simulink model "m02_PMSM_HDL"  (R2023b)
settings: Solver=FixedStepDiscrete  StartTime=0.0  StopTime=0.6  RelTol=1e-3  AbsTol=1e-3
PreLoadFcn:
  | control_data;
  | pmsm_data;
  | 
  | avgFactor = 1;
undefined symbols (not defined in the file): ee_sli_rtmsupport, f1478573793584, f1859323186544, fsw, gcbh, J, Ld, Lq, N, PM, Pmax, Tmax, Ts, Tsc
libraries: hdlssclib x24, simulink x8, SimscapeFPGAHIL_lib x6, fpga_utils_lib x5, hdlsllib x4, eeTransforms x2, eePwmGeneratorTwoLevel x1, eePmsmCurrentController x1, eePmsmCurrentReferenceGen x1, eeVelocityController x1
(part 1 of 3)
Description:
  | Three-Phase PMSM Drive
settings Model: DataTypeOverride=Off  SimulationMode=accelerator  Creator=The MathWorks, Inc.  LastModifiedBy=promero
settings SolverCC: AutoScaleAbsTol=off  MaxConsecutiveMinStep=2  ZeroCrossAlgorithm=Adaptive  AlgebraicLoopSolver=TrustRegion  MaxZcPerStep=1
settings DataIOCC: MaxDataPoints=690000  SaveOutput=off  DSMLogging=off  SaveTime=off
settings OptimizationCC: BlockReduction=off  ConditionallyExecuteInputs=off  DefaultParameterBehavior=Inlined  InheritOutputTypeSmallerThanSingle=on  ReuseModelBlockBuffer=off  LifeSpan=inf
settings DebuggingCC: AlgebraicLoopMsg=error  UnderspecifiedInitializationDetection=Classic  MergeDetectMultiDrivingBlocksExec=none  MaxConsecutiveZCsMsg=none  IgnoredZcDiagnostic=none  InheritedTsInSrcMsg=none  SingleTaskRateTransMsg=error  UnconnectedInputMsg=warning  UnconnectedOutputMsg=warning  UnconnectedLineMsg=warning  AllowSymbolicDim=off  PregeneratedLibrarySubsystemCodeDiagnostic=none  SFUnexpectedBacktrackingDiag=warning  SFNoUnconditionalDefaultTransitionDiag=warning  SFExecutionAtInitializationDiag=none  ArithmeticOperatorsInVariantConditions=warning
settings HardwareCC: ProdBitPerPointer=32  ProdBitPerSizeT=32  ProdBitPerPtrDiffT=32  ProdLargestAtomicFloat=None  ProdIntDivRoundTo=Undefined  ProdEndianess=Unspecified  ProdWordSize=32  ProdHWDeviceType=ASIC/FPGA->ASIC/FPGA  TargetBitPerPointer=64  TargetBitPerSizeT=64  TargetBitPerPtrDiffT=64  TargetLongLongMode=on  TargetIntDivRoundTo=Zero  TargetEndianess=LittleEndian  TargetWordSize=64  TargetHWDeviceType=Custom Processor->MATLAB Host Computer  ProdEqTarget=off
settings ModelReferenceCC: EnableRefExpFcnMdlSchedulingChecks=on  PropagateSignalLabelsOutOfModel=off
settings SFSimCC: SimUseLocalCustomCode=off
settings RTWCC: RTWUseLocalCustomCode=off  DLArmComputeVersion=19.05
settings CodeAppCC: StateflowObjectComments=on
settings GRTTargetCC: TargetLangStandard=C89/C90 (ANSI)
settings ConfigComp: CovMetricSettings=dw  CovSaveCumulativeToWorkspaceVar=on  CovSaveSingleToWorkspaceVar=on  CovExternalEMLEnable=off  CovSFcnEnable=off
settings SimscapeCC: SimscapeLogSimulationStatistics=on  SimscapeLogName=simlog_ee_pmsm_drive  SimscapeLogDataHistory=690000

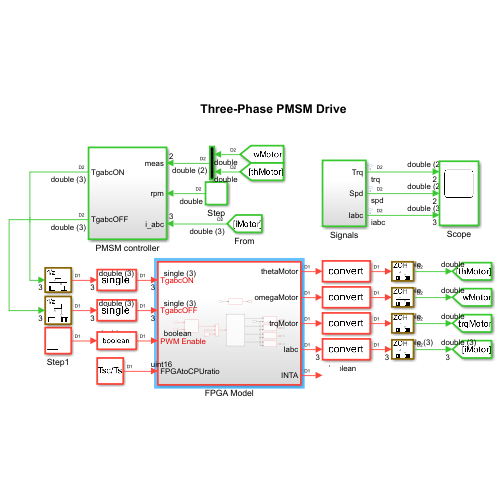
[thumbnail: Simulink's stored preview of the top-level diagram]
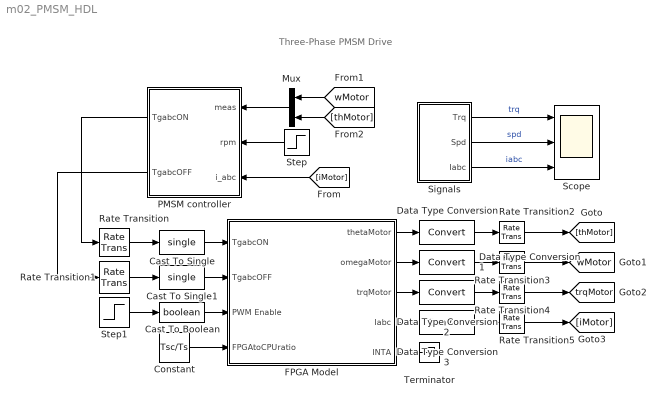
== system m02_PMSM_HDL ==
  note: Three-Phase PMSM Drive
  Cast To Boolean : DataTypeConversion  OutDataTypeStr=boolean  SaturateOnIntegerOverflow=off  RndMeth=Floor
  Cast To Single : DataTypeConversion  OutDataTypeStr=single  SaturateOnIntegerOverflow=off  RndMeth=Floor
  Cast To Single1 : DataTypeConversion  OutDataTypeStr=single  SaturateOnIntegerOverflow=off  RndMeth=Floor
  Constant : Constant  Value=Tsc/Ts  OutDataTypeStr=uint16  SampleTime=-1
  Data Type Conversion{,1..3} (4 alike) : DataTypeConversion  SaturateOnIntegerOverflow=off  RndMeth=Floor
  FPGA Model : Subsystem
  Mux : Mux  Inputs=2
  PMSM controller : Subsystem
  Rate Transition : RateTransition  OutPortSampleTime=Ts
  Rate Transition1 : RateTransition  OutPortSampleTime=Ts
  Rate Transition{2..5} (4 alike) : RateTransition  OutPortSampleTime=Tsc
  Scope : Scope  NumInputPorts=3
  "Signals " : Subsystem
  Step : Step  Time=0.1  After=500  SampleTime=Tsc
  Step1 : Step  Time=1e-4
  Terminator : Terminator
  tag scope: trqMotor=global, wMotor=global
  wires:
  "Signals "/2(Spd) -> Scope/2  "spd"
  "Signals "/1(Trq) -> Scope/1  "trq"
  "Signals "/3(Iabc) -> Scope/3  "iabc"
  Step/1 -> PMSM controller/2(rpm)
  Mux/1 -> PMSM controller/1(meas)
  [iMotor] -> PMSM controller/3(i_abc)
  PMSM controller/1(TgabcON) -> Rate Transition/1
  PMSM controller/2(TgabcOFF) -> Rate Transition1/1
  Step1/1 -> Cast To Boolean/1
  FPGA Model/1(thetaMotor) -> Data Type Conversion/1
  FPGA Model/2(omegaMotor) -> Data Type Conversion1/1
  FPGA Model/3(trqMotor) -> Data Type Conversion2/1
  FPGA Model/4(Iabc) -> Data Type Conversion3/1
  Data Type Conversion2/1 -> Rate Transition4/1
  Data Type Conversion3/1 -> Rate Transition5/1
  Data Type Conversion1/1 -> Rate Transition3/1
  Data Type Conversion/1 -> Rate Transition2/1
  [wMotor] -> Mux/1
  [thMotor] -> Mux/2
  Cast To Single/1 -> FPGA Model/1(TgabcON)
  Cast To Single1/1 -> FPGA Model/2(TgabcOFF)
  Cast To Boolean/1 -> FPGA Model/3(PWM Enable)
  Rate Transition/1 -> Cast To Single/1
  Rate Transition1/1 -> Cast To Single1/1
  Rate Transition2/1 -> [thMotor]
  Rate Transition3/1 -> [wMotor]
  Rate Transition4/1 -> [trqMotor]
  Rate Transition5/1 -> [iMotor]
  Constant/1 -> FPGA Model/4(FPGAtoCPUratio)
  FPGA Model/5(INTA) -> Terminator/1

== system m02_PMSM_HDL/FPGA Model ==
  TgabcON : Inport
  TgabcOFF : Inport  Port=2
  PWM Enable : Inport  Port=3
  FPGAtoCPUratio : Inport  Port=4
  Constant : Constant  Value=[0,1,0,1,0,1]  OutDataTypeStr=boolean  SampleTime=-1
  FPGAtoCPUratio1 : InportShadow  Port=4
  HDL Moving Average Tunable{,1..3} (4 alike) : fpga_utils_lib/HDL Moving Average Tunable  SystemSampleTime=-1  VariantActivationTime=update diagram  AllowFlexibleInterface=on  Latency=0  AutoFrameSizeCalculation=off
  HDL Plant : Subsystem  Variant=on  VariantControlMode=label  VariantControl=Pejovic HDL Plant  LabelModeActiveChoice=Pejovic
  Interrupt : fpga_utils_lib/Interrupt  SystemSampleTime=-1  VariantActivationTime=update diagram  AllowFlexibleInterface=on  Latency=0  AutoFrameSizeCalculation=off
  PWM Gate Signal Generator : Subsystem  Variant=on  VariantControlMode=label  VariantControl=Choice  LabelModeActiveChoice=hdlVar
  Switch : Switch  Criteria=u2 ~= 0  SaturateOnIntegerOverflow=off
  thetaMotor : Outport  OutDataTypeStr=single
  omegaMotor : Outport  Port=2  OutDataTypeStr=single
  trqMotor : Outport  Port=3  OutDataTypeStr=single
  Iabc : Outport  Port=4  OutDataTypeStr=single
  INTA : Outport  Port=5
  wires:
  Constant/1 -> Switch/3
  PWM Enable/1 -> Switch/2
  TgabcON/1 -> PWM Gate Signal Generator/1(TgabcON)
  TgabcOFF/1 -> PWM Gate Signal Generator/2(TgabcOFF)
  PWM Gate Signal Generator/1(g) -> Switch/1
  HDL Moving Average Tunable/1 -> thetaMotor/1
  HDL Moving Average Tunable1/1 -> omegaMotor/1
  HDL Moving Average Tunable2/1 -> trqMotor/1
  HDL Moving Average Tunable3/1 -> Iabc/1
  FPGAtoCPUratio/1 -> HDL Moving Average Tunable3/2, HDL Moving Average Tunable2/2, HDL Moving Average Tunable1/2, HDL Moving Average Tunable/2
  Interrupt/1 -> INTA/1
  FPGAtoCPUratio1/1 -> Interrupt/1
  Switch/1 -> HDL Plant/1(In1)
  HDL Plant/1(thetaMotor) -> HDL Moving Average Tunable/1
  HDL Plant/2(omegaMotor) -> HDL Moving Average Tunable1/1
  HDL Plant/3(trqMotor) -> HDL Moving Average Tunable2/1
  HDL Plant/4(Iabc) -> HDL Moving Average Tunable3/1

== system m02_PMSM_HDL/PMSM controller ==
  meas : Inport
  rpm : Inport  Port=2
  i_abc : Inport  Port=3
  Bus Selector : BusSelector  OutputSignals=iabc [A],Reference,TqRef [N*m]
  Demux1 : Demux  Outputs=2
  PMSM Field-Oriented Control : Subsystem  AncestorBlock=eePmsmFieldOrientedControl/PMSM Field-Oriented Control  LoadFcn=ee_sli_rtmsupport( 'loadfcn', gcbh );  mask(PMSM Field-Oriented Control){winding_type=Wye-wound, CtrlMode=Velocity control, Vnom=48, Pmax=Pmax, Tmax=Tmax*1.5, p=N, Vdc_on=10, Ts=Ts, Tsc=Tsc, CtrlType=PI control, Kp_w=60, Ki_w=300*2, Kv_w=1, Kaw_w=1000, RefType=Zero d-axis control, rpmVec=[0, 3000], TqVec=[-100, 0, 100], VdcVec=[300, 350], PWMMode=SPWM: sinusoidal PWM, ModFactor=1, idMatrix=zeros(2,3,2), iqMatrix=zeros(2,3,2), psim=PM, Ld=0.00024, Lq=0.00029, Rs=0.01, AxisAlignment=Q-axis, Kp_id=0.1, Ki_id=10, Kaw_id=1000, Kp_iq=0.1, Ki_iq=10, Kaw_iq=1000, AxisPrio=Q-axis, ActZC=off, ActFF=on, ParamTypeFF=Constant parameters, LdFF=Ld, LqFF=Lq, psimFF=PM, idVect=[-200, 0, 200], iqVect=[-200, 0, 200], LdMatrix=0.0002 * ones(3, 3), LqMatrix=0.0002 * ones(3, 3), psimMatrix=0.04 * ones(3, 3), CPWMMode=SPWM: sinusoidal PWM, SamplingMode=Natural, fsw=fsw}
      mask prompts: winding_type "physmod:ee:library:comments:control:eePmsmFieldOrientedControl:WindingType_MP"; CtrlMode "physmod:ee:library:comments:control:eePmsmFieldOrientedControl:ControlMode_MP"; Vnom "physmod:ee:library:comments:control:eePmsmFieldOrientedControl:NominalDclinkVoltageV_MP"; Pmax "physmod:ee:library:comments:control:eePmsmFieldOrientedControl:MaximumPowerW_MP"; Tmax "physmod:ee:library:comments:control:eePmsmFieldOrientedControl:MaximumTorqueNm_MP"; p "physmod:ee:library:comments:control:eePmsmFieldOrientedControl:NumberOfRotorPolePairs_MP"; Vdc_on "physmod:ee:library:comments:control:eePmsmFieldOrientedControl:InverterDclinkVoltageThresholdV_MP"; Ts "physmod:ee:library:comments:control:eePmsmFieldOrientedControl:FundamentalSampleTimes_MP"; Tsc "physmod:ee:library:comments:control:eePmsmFieldOrientedControl:ControlSampleTimes_MP"; CtrlType "physmod:ee:library:comments:control:eePmsmFieldOrientedControl:ControlType_MP"; Kp_w "physmod:ee:library:comments:control:eePmsmFieldOrientedControl:ControllerProportionalGain_MP"; Ki_w "physmod:ee:library:comments:control:eePmsmFieldOrientedControl:ControllerIntegralGain_MP"; Kv_w "physmod:ee:library:comments:control:eePmsmFieldOrientedControl:PControllerProportionalGain_MP"; Kaw_w "physmod:ee:library:comments:control:eePmsmFieldOrientedControl:IntegralAntiwindupGain_MP"; RefType "physmod:ee:library:comments:control:eePmsmFieldOrientedControl:CurrentReferences_MP"; rpmVec "physmod:ee:library:comments:control:eePmsmFieldOrientedControl:MechanicalSpeedVectorWMechanicalrpm_MP"; TqVec "physmod:ee:library:comments:control:eePmsmFieldOrientedControl:TorqueReferenceVectorTqRefNm_MP"; VdcVec "physmod:ee:library:comments:control:eePmsmFieldOrientedControl:DClinkVoltageVectorVdcV_MP"; PWMMode "physmod:ee:library:comments:control:eePmsmCurrentReferenceGen:PWMMethod_MP"; ModFactor "physmod:ee:library:comments:control:eePmsmCurrentReferenceGen:ModulationFactor_MP"; idMatrix "physmod:ee:library:comments:control:eePmsmFieldOrientedControl:DaxisCurrentReferenceMatrixIdwMechanicalTqRefVdcA_MP"; iqMatrix "physmod:ee:library:comments:control:eePmsmFieldOrientedControl:QaxisCurrentReferenceMatrixIqwMechanicalTqRefVdcA_MP"; psim "physmod:ee:library:comments:control:eePmsmFieldOrientedControl:PermanentMagnetFluxLinkageWb_MP"; Ld "physmod:ee:library:comments:control:eePmsmFieldOrientedControl:DaxisInductanceH_MP"; Lq "physmod:ee:library:comments:control:eePmsmFieldOrientedControl:QaxisInductanceH_MP"; Rs "physmod:ee:library:comments:control:eePmsmFieldOrientedControl:StatorResistanceOhm_MP"; AxisAlignment "physmod:ee:library:comments:control:eePmsmFieldOrientedControl:PhaseaAxisAlignment_MP"; Kp_id "physmod:ee:library:comments:control:eePmsmFieldOrientedControl:DaxisCurrentProportionalGain_MP"; Ki_id "physmod:ee:library:comments:control:eePmsmFieldOrientedControl:DaxisCurrentIntegralGain_MP"; Kaw_id "physmod:ee:library:comments:control:eePmsmFieldOrientedControl:DaxisCurrentAntiwindupGain_MP"; Kp_iq "physmod:ee:library:comments:control:eePmsmFieldOrientedControl:QaxisCurrentProportionalGain_MP"; Ki_iq "physmod:ee:library:comments:control:eePmsmFieldOrientedControl:QaxisCurrentIntegralGain_MP"; Kaw_iq "physmod:ee:library:comments:control:eePmsmFieldOrientedControl:QaxisCurrentAntiwindupGain_MP"; AxisPrio "physmod:ee:library:comments:control:eePmsmFieldOrientedControl:AxisPrioritization_MP"; ActZC "physmod:ee:library:comments:control:eePmsmFieldOrientedControl:EnableZeroCancellation_MP"; ActFF "physmod:ee:library:comments:control:eePmsmFieldOrientedControl:EnablePrecontrolVoltage_MP"; ParamTypeFF "physmod:ee:library:comments:control:eePmsmFieldOrientedControl:MachineParameters_MP"; LdFF "physmod:ee:library:comments:control:eePmsmFieldOrientedControl:DaxisInductanceForFeedforwardPrecontrolH_MP"; LqFF "physmod:ee:library:comments:control:eePmsmFieldOrientedControl:QaxisInductanceForFeedforwardPrecontrolH_MP"; psimFF "physmod:ee:library:comments:control:eePmsmFieldOrientedControl:PermanentMagnetFluxLinkageForFeedforwardPrecontrolWb_MP"; idVect "physmod:ee:library:comments:control:eePmsmFieldOrientedControl:DaxisCurrentVectorIdA_MP"; iqVect "physmod:ee:library:comments:control:eePmsmFieldOrientedControl:QaxisCurrentVectorIqA_MP"; LdMatrix "physmod:ee:library:comments:control:eePmsmFieldOrientedControl:LdMatrixLdidiqH_MP"; LqMatrix "physmod:ee:library:comments:control:eePmsmFieldOrientedControl:LqMatrixLqidiqH_MP"; psimMatrix "physmod:ee:library:comments:control:eePmsmFieldOrientedControl:PermanentMagnetFluxLinkageMatrixPMidiqWb_MP"; CPWMMode "physmod:ee:library:comments:control:eePmsmFieldOrientedControl:PWMMethod_MP"; SamplingMode "physmod:ee:library:comments:control:eePmsmFieldOrientedControl:SamplingMode_MP"; fsw "physmod:ee:library:comments:control:eePmsmFieldOrientedControl:SwitchingFrequencyHz_MP"
      mask help: physmod:ee:library:comments:control:eePmsmFieldOrientedControl:PMSMFieldOrientedControl_MD
      mask init:
      | if ParamTypeFF == 1
      |     idVect = [-200, 200];
      |     iqVect = [-200, 200];
      |     LdMatrix = LdFF*ones(2, 2);
      |     LqMatrix = LqFF*ones(2, 2);
      |     psimMatrix = psimFF*ones(2, 2);
      | end
      | 
      | switch winding_type
      |     case 1
      |         theta_offset = 0;
      |     case 2
      |         theta_offset = -(120/p)*pi/180;
      |     otherwise
      |         theta_offset = 0;
      | end
      | 
      | switch CPWMMode
      |     case 'SPWM: sinusoidal PWM'
      |         set_param(gcb,'PWMMode','SPWM: sinusoidal PWM');
      |     case 'SVM: space vector modulation'
      |         set_param(gcb,'PWMMode','SVM: space vector modulation')
      | end
      settings: CopyFcn=ee_sli_rtmsupport( 'copyfcn', gcbh );  DeleteFcn=ee_sli_rtmsupport( 'deletefcn', gcbh );  ModelCloseFcn=ee_sli_rtmsupport( 'modelclosefcn', gcbh );  PostSaveFcn=ee_sli_rtmsupport( 'postsavefcn', gcbh );  PreCopyFcn=ee_sli_rtmsupport( 'precopyfcn', gcbh );  OpenFcn=ee_sli_rtmsupport( 'openfcn', gcbh );  CloseFcn=ee_sli_rtmsupport( 'closefcn', gcbh );  PreDeleteFcn=ee_sli_rtmsupport( 'predeletefcn', gcbh );
      mask Help: web(nesl_help(gcbh))
      mask TypeOptions winding_type: physmod:ee:library:comments:control:eePmsmFieldOrientedControl:WyeWound_PV | physmod:ee:library:comments:control:eePmsmFieldOrientedControl:DeltaWound_PV
      mask Callback winding_type: ee.mask.callbackPopupPmsmFoc(gcb);
      mask TypeOptions CtrlMode: physmod:ee:library:comments:control:eePmsmFieldOrientedControl:VelocityControl_PV | physmod:ee:library:comments:control:eePmsmFieldOrientedControl:TorqueControl_PV
      mask Callback CtrlMode: ee.mask.callbackPopupPmsmFoc(gcb);
      mask TypeOptions Vnom:
      | Outer loop control/PMSM Current Reference
      | Generator/Vnom
      mask TypeOptions Pmax:
      | Outer loop control/PMSM Current Reference
      | Generator/Pmax
      mask TypeOptions Tmax:
      | Outer loop control/PMSM Current Reference
      | Generator/Tmax
      mask TypeOptions CtrlType: Outer loop control/Velocity Controller/CtrlType
      mask Callback CtrlType: ee.mask.callbackPopupPmsmFoc(gcb);
      mask TypeOptions Kp_w: Outer loop control/Velocity Controller/Kp_w
      mask TypeOptions Ki_w: Outer loop control/Velocity Controller/Ki_w
      mask TypeOptions Kv_w: Outer loop control/Velocity Controller/Kv_w
      mask TypeOptions Kaw_w: Outer loop control/Velocity Controller/Kaw_w
      mask TypeOptions RefType:
      | Outer loop control/PMSM Current Reference
      | Generator/RefType
      mask Callback RefType: ee.mask.callbackPopupPmsmFoc(gcb);
      mask TypeOptions rpmVec:
      | Outer loop control/PMSM Current Reference
      | Generator/rpmVec
      mask TypeOptions TqVec:
      | Outer loop control/PMSM Current Reference
      | Generator/TqVec
      mask TypeOptions VdcVec:
      | Outer loop control/PMSM Current Reference
      | Generator/VdcVec
      mask TypeOptions PWMMode:
      | Outer loop control/PMSM Current Reference
      | Generator/PWMMode
      mask TypeOptions ModFactor:
      | Outer loop control/PMSM Current Reference
      | Generator/ModFactor
      mask TypeOptions idMatrix:
      | Outer loop control/PMSM Current Reference
      | Generator/idMatrix
      mask TypeOptions iqMatrix:
      | Outer loop control/PMSM Current Reference
      | Generator/iqMatrix
      mask TypeOptions psim:
      | Outer loop control/PMSM Current Reference
      | Generator/psim
      mask TypeOptions Ld:
      | Outer loop control/PMSM Current Reference
      | Generator/Ld
      mask TypeOptions Lq:
      | Outer loop control/PMSM Current Reference
      | Generator/Lq
      mask TypeOptions Rs:
      | Outer loop control/PMSM Current Reference
      | Generator/Rs
      mask TypeOptions AxisAlignment: Inner loop control/Park Transform/AxisAlignment
      mask TypeOptions Kp_id:
      | Inner loop control/PMSM Current Controller
      | with Pre-Control/Kp_id
      mask TypeOptions Ki_id:
      | Inner loop control/PMSM Current Controller
      | with Pre-Control/Ki_id
      mask TypeOptions Kaw_id:
      | Inner loop control/PMSM Current Controller
      | with Pre-Control/Kaw_id
      mask TypeOptions Kp_iq:
      | Inner loop control/PMSM Current Controller
      | with Pre-Control/Kp_iq
      mask TypeOptions Ki_iq:
      | Inner loop control/PMSM Current Controller
      | with Pre-Control/Ki_iq
      mask TypeOptions Kaw_iq:
      | Inner loop control/PMSM Current Controller
      | with Pre-Control/Kaw_iq
      mask TypeOptions AxisPrio:
      | Inner loop control/PMSM Current Controller
      | with Pre-Control/AxisPrio
      mask TypeOptions ActZC:
      | Inner loop control/PMSM Current Controller
      | with Pre-Control/ActZC
      mask TypeOptions ActFF:
      | Inner loop control/PMSM Current Controller
      | with Pre-Control/ActFF
      mask Callback ActFF: ee.mask.callbackPopupPmsmFoc(gcb);
      mask TypeOptions ParamTypeFF: physmod:ee:library:comments:control:eePmsmFieldOrientedControl:ConstantParameters_PV | physmod:ee:library:comments:control:eePmsmFieldOrientedControl:LookupTableBasedParameters_PV
      mask Callback ParamTypeFF: ee.mask.callbackPopupPmsmFoc(gcb);
      mask TypeOptions idVect:
      | Inner loop control/PMSM Current Controller
      | with Pre-Control/idVect
      mask TypeOptions iqVect:
      | Inner loop control/PMSM Current Controller
      | with Pre-Control/iqVect
      mask TypeOptions LdMatrix:
      | Inner loop control/PMSM Current Controller
      | with Pre-Control/LdMatrix
      mask TypeOptions LqMatrix:
      | Inner loop control/PMSM Current Controller
      | with Pre-Control/LqMatrix
      mask TypeOptions psimMatrix:
      | Inner loop control/PMSM Current Controller
      | with Pre-Control/psimMatrix
      mask TypeOptions CPWMMode:
      | PWM/PWM Generator
      | (Three-phase, Two-level)/CPWMMode
      mask TypeOptions SamplingMode:
      | PWM/PWM Generator
      | (Three-phase, Two-level)/SamplingMode
      mask DialogControl Container4 Prompt: physmod:ee:library:comments:control:eePmsmFieldOrientedControl:tab_General
      mask DialogControl winding_type Prompt: Winding type
      mask DialogControl CtrlMode Prompt: Control mode
      mask DialogControl Vnom Prompt: Nominal dc-link voltage (V)
      mask DialogControl Pmax Prompt: Maximum power (W)
      mask DialogControl Tmax Prompt: Maximum torque (N*m)
      mask DialogControl p Prompt: Number of rotor pole pairs
      mask DialogControl Vdc_on Prompt: Inverter dc-link voltage threshold (V)
      mask DialogControl Ts Prompt: Fundamental sample time (s)
      mask DialogControl Tsc Prompt: Control sample time (s)
      mask DialogControl Container7 Prompt: physmod:ee:library:comments:control:eePmsmFieldOrientedControl:tab_OuterLoop
      mask DialogControl CtrlType Prompt: Control type
      mask DialogControl Kp_w Prompt: Controller proportional gain
      mask DialogControl Ki_w Prompt: Controller integral gain
      mask DialogControl Kv_w Prompt: P controller proportional gain
      mask DialogControl Kaw_w Prompt: Integral anti-windup gain
      mask DialogControl RefType Prompt: Current references
      mask DialogControl rpmVec Prompt: Mechanical speed vector, wMechanical (rpm)
      mask DialogControl TqVec Prompt: Torque reference vector, TqRef (N*m)
      mask DialogControl VdcVec Prompt: DC-link voltage vector, Vdc (V)
      mask DialogControl PWMMode Prompt: PWM method
      mask DialogControl ModFactor Prompt: Modulation factor
      mask DialogControl idMatrix Prompt: D-axis current reference matrix, id(wMechanical,TqRef,Vdc), (A)
      mask DialogControl iqMatrix Prompt: Q-axis current reference matrix, iq(wMechanical,TqRef,Vdc), (A)
      mask DialogControl psim Prompt: Permanent magnet flux linkage (Wb)
      mask DialogControl Ld Prompt: D-axis inductance (H)
      mask DialogControl Lq Prompt: Q-axis inductance (H)
      mask DialogControl Rs Prompt: Stator resistance (Ohm)
      mask DialogControl Container8 Prompt: physmod:ee:library:comments:control:eePmsmFieldOrientedControl:tab_InnerLoop
      mask DialogControl AxisAlignment Prompt: Phase-a axis alignment
      mask DialogControl Kp_id Prompt: D-axis current proportional gain
      mask DialogControl Ki_id Prompt: D-axis current integral gain
      mask DialogControl Kaw_id Prompt: D-axis current anti-windup gain
      mask DialogControl Kp_iq Prompt: Q-axis current proportional gain
      mask DialogControl Ki_iq Prompt: Q-axis current integral gain
      mask DialogControl Kaw_iq Prompt: Q-axis current anti-windup gain
      mask DialogControl AxisPrio Prompt: Axis prioritization
      mask DialogControl ActZC Prompt: Enable zero cancellation
      mask DialogControl ActFF Prompt: Enable pre-control voltage
      mask DialogControl ParamTypeFF Prompt: Machine parameters
      mask DialogControl LdFF Prompt: D-axis inductance for feed-forward pre-control (H)
      mask DialogControl LqFF Prompt: Q-axis inductance for feed-forward pre-control (H)
      mask DialogControl psimFF Prompt: Permanent magnet flux linkage for feed-forward pre-control (Wb)
      mask DialogControl idVect Prompt: D-axis current vector, id (A)
      mask DialogControl iqVect Prompt: Q-axis current vector, iq (A)
      mask DialogControl LdMatrix Prompt: Ld matrix, Ld(id,iq), (H)
      mask DialogControl LqMatrix Prompt: Lq matrix, Lq(id,iq), (H)
      mask DialogControl psimMatrix Prompt: Permanent magnet flux linkage matrix, PM(id,iq), (Wb)
      mask DialogControl Container9 Prompt: physmod:ee:library:comments:control:eePmsmFieldOrientedControl:tab_PWM
      mask DialogControl CPWMMode Prompt: PWM method
      mask DialogControl SamplingMode Prompt: Sampling mode
      mask DialogControl fsw Prompt: Switching frequency (Hz)
  Rate Limiter : RateLimiter  RisingSlewLimit=Tmax/J  FallingSlewLimit=-Tmax/J  SampleTimeMode=inherited
  Vdc : Constant  Value=48  SampleTime=Tsc
  "rpm -> rad/s [mech.]" : Gain  Gain=2*pi/60
  TgabcON : Outport
  TgabcOFF : Outport  Port=2
  tag scope: iMotor=global, trqDemand=global, wDemand=global
  wires:
  Vdc/1 -> PMSM Field-Oriented Control/5(vdcSens)
  PMSM Field-Oriented Control/3(Visualization) -> Bus Selector/1
  i_abc/1 -> PMSM Field-Oriented Control/2(iabcSens)
  meas/1 -> Demux1/1
  Demux1/1 -> PMSM Field-Oriented Control/3(wSens)
  Demux1/2 -> PMSM Field-Oriented Control/4(thSens)
  Bus Selector/1 -> [iMotor]  "<iabc [A]>"
  Bus Selector/2 -> [wDemand]  "<Reference>"
  Bus Selector/3 -> [trqDemand]  "<TqRef [N*m]>"
  rpm/1 -> "rpm -> rad/s [mech.]"/1
  Rate Limiter/1 -> PMSM Field-Oriented Control/1(Reference)
  "rpm -> rad/s [mech.]"/1 -> Rate Limiter/1
  PMSM Field-Oriented Control/1(TgabcON) -> TgabcON/1
  PMSM Field-Oriented Control/2(TgabcOFF) -> TgabcOFF/1

== system m02_PMSM_HDL/Signals  ==
  Mux : Mux  Inputs=2
  Mux1 : Mux  Inputs=2
  RT4 : RateTransition  OutPortSampleTime=Tsc
  RT5 : RateTransition  OutPortSampleTime=Tsc
  rad/s2rpm : Gain  Gain=60/(2*pi)
  Trq : Outport  VectorParamsAs1DForOutWhenUnconnected=off
  Spd : Outport  Port=2  VectorParamsAs1DForOutWhenUnconnected=off
  Iabc : Outport  Port=3  VectorParamsAs1DForOutWhenUnconnected=off
  wires:
  [trqDemand] -> Mux/1
  Mux1/1 -> rad/s2rpm/1
  Mux/1 -> Trq/1  "Torque"
  [iMotor] -> Iabc/1  "Currents"
  [wDemand] -> Mux1/1
  rad/s2rpm/1 -> Spd/1  "Speed"
  [trqMotor] -> RT4/1
  [wMotor] -> RT5/1
  RT4/1 -> Mux/2
  RT5/1 -> Mux1/2

== system m02_PMSM_HDL/FPGA Model/HDL Plant ==
  In1 : Inport
  Pejovic HDL Plant : Subsystem  InitFcn=load('f1478573793584.mat');  VariantControl=Pejovic
  Standard HDL Plant : Subsystem  InitFcn=load('f1859323186544.mat');  VariantControl=Standard
  thetaMotor : Outport
  omegaMotor : Outport  Port=2
  trqMotor : Outport  Port=3
  Iabc : Outport  Port=4

== system m02_PMSM_HDL/FPGA Model/PWM Gate Signal Generator ==
  TgabcON : Inport
  TgabcOFF : Inport  Port=2
  HDL counter : Subsystem  VariantControl=hdlVar
      settings: LibrarySourceBlock=|
      | ee_sl_lib/Pulse Width
      | Modulation/PWM Gate Signal Generator
      | (Three-phase, Two-level)
  Off-the-shelf block : eePwmGeneratorTwoLevel/PWM Gate Signal Generator (Three-phase, Two-level)  VariantControl=defVar  fsw=fsw  Ts=Ts
      settings: SamplingMode=Natural
      settings: LibrarySourceBlock=|
      | ee_sl_lib/Pulse Width
      | Modulation/PWM Gate Signal Generator
      | (Three-phase, Two-level)
  g : Outport

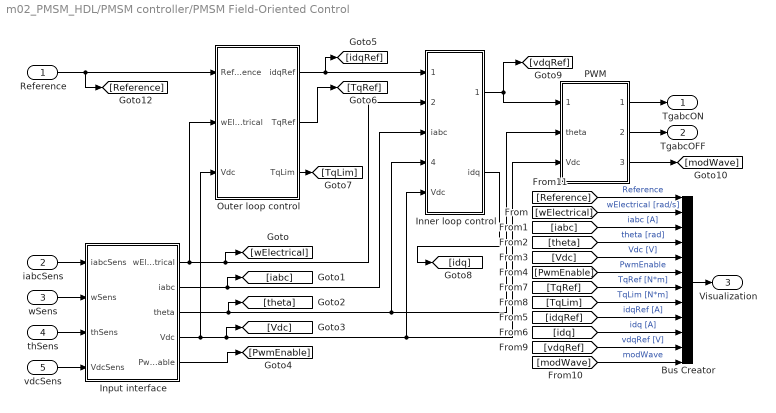
== system m02_PMSM_HDL/PMSM controller/PMSM Field-Oriented Control ==
  Reference : Inport  SampleTime=Tsc
  iabcSens : Inport  Port=2  SampleTime=Tsc
  wSens : Inport  Port=3  SampleTime=Tsc
  thSens : Inport  Port=4  SampleTime=Tsc
  vdcSens : Inport  Port=5  SampleTime=Tsc
  Bus Creator : BusCreator  Inputs=12
  Inner loop control : Subsystem
  Input interface : Subsystem
  Outer loop control : Subsystem
  PWM : Subsystem
  TgabcON : Outport
  TgabcOFF : Outport  Port=2
  Visualization : Outport  Port=3  VectorParamsAs1DForOutWhenUnconnected=off
  wires:
  [modWave] -> Bus Creator/12  "modWave"
  [vdqRef] -> Bus Creator/11  "vdqRef [V]"
  [idq] -> Bus Creator/10  "idq [A]"
  [idqRef] -> Bus Creator/9  "idqRef [A]"
  [TqLim] -> Bus Creator/8  "TqLim [N*m]"
  [TqRef] -> Bus Creator/7  "TqRef [N*m]"
  [PwmEnable] -> Bus Creator/6  "PwmEnable"
  [Vdc] -> Bus Creator/5  "Vdc [V]"
  [theta] -> Bus Creator/4  "theta [rad]"
  [iabc] -> Bus Creator/3  "iabc [A]"
  [wElectrical] -> Bus Creator/2  "wElectrical [rad/s]"
  [Reference] -> Bus Creator/1  "Reference"
  PWM/3(ModWave) -> [modWave]
  Inner loop control/2(idq) -> [idq]
  Outer loop control/3(TqLim) -> [TqLim]
  Outer loop control/2(TqRef) -> [TqRef]
  Bus Creator/1 -> Visualization/1
  Input interface/5(PwmEnable) -> [PwmEnable]
  Inner loop control/1(vdqRef) -> PWM/1(vdqRef), [vdqRef]
  Input interface/1(wElectrical) -> Outer loop control/2(wElectrical), Inner loop control/2(wElectrical), [wElectrical]
  Input interface/4(Vdc) -> Outer loop control/3(Vdc), Inner loop control/5(Vdc), PWM/3(Vdc), [Vdc]
  Reference/1 -> Outer loop control/1(Reference), [Reference]
  vdcSens/1 -> Input interface/4(VdcSens)
  thSens/1 -> Input interface/3(thSens)
  wSens/1 -> Input interface/2(wSens)
  iabcSens/1 -> Input interface/1(iabcSens)
  Outer loop control/1(idqRef) -> Inner loop control/1(idq_ref), [idqRef]
  Input interface/3(theta) -> Inner loop control/4(theta), PWM/2(theta), [theta]
  Input interface/2(iabc) -> Inner loop control/3(iabc), [iabc]
  PWM/2(TgabcOFF) -> TgabcOFF/1
  PWM/1(TgabcON) -> TgabcON/1

== system m02_PMSM_HDL/FPGA Model/HDL Plant/Pejovic HDL Plant ==
  In1 : Inport
  Controller{,1..5} (6 alike) : SimscapeFPGAHIL_lib/Linearized Switch Models/Switch/Controller  threshold=0.5  Gs=1e-6  s=1  avgFactor=avgFactor  isFixedPoint=off
  Demux : Demux  Outputs=6
  HDL Subsystem : Subsystem
  Signal Specification : SignalSpecification  OutDataTypeStr=boolean
  thetaMotor : Outport
  omegaMotor : Outport  Port=2
  trqMotor : Outport  Port=3
  Iabc : Outport  Port=4
  wires:
  HDL Subsystem/15(vs_in6) -> Controller2/1  "vs_in6"
  Demux/6 -> Controller2/3
  In1/1 -> Signal Specification/1
  HDL Subsystem/12(is_in5) -> Controller5/2  "is_in5"
  HDL Subsystem/10(is_in4) -> Controller1/2  "is_in4"
  HDL Subsystem/9(vs_in3) -> Controller4/1  "vs_in3"
  Controller3/1 -> HDL Subsystem/4(ic_out1)
  Demux/4 -> Controller1/3
  Demux/2 -> Controller/3
  HDL Subsystem/13(vs_in5) -> Controller5/1  "vs_in5"
  HDL Subsystem/4(is_in1) -> Controller3/2  "is_in1"
  Controller5/1 -> HDL Subsystem/6(ic_out5)
  Demux/3 -> Controller4/3
  Demux/5 -> Controller5/3
  Controller2/1 -> HDL Subsystem/3(ic_out6)
  HDL Subsystem/3(trqMotor) -> trqMotor/1  "trqMotor"
  Demux/1 -> Controller3/3
  HDL Subsystem/5(vs_in1) -> Controller3/1  "vs_in1"
  HDL Subsystem/11(vs_in4) -> Controller1/1  "vs_in4"
  HDL Subsystem/14(is_in6) -> Controller2/2  "is_in6"
  Controller/1 -> HDL Subsystem/1(ic_out2)
  HDL Subsystem/8(is_in3) -> Controller4/2  "is_in3"
  HDL Subsystem/2(omegaMotor) -> omegaMotor/1  "omegaMotor"
  Controller4/1 -> HDL Subsystem/5(ic_out3)
  HDL Subsystem/7(vs_in2) -> Controller/1  "vs_in2"
  HDL Subsystem/6(is_in2) -> Controller/2  "is_in2"
  Controller1/1 -> HDL Subsystem/2(ic_out4)
  Signal Specification/1 -> Demux/1
  HDL Subsystem/1(thetaMotor) -> thetaMotor/1  "thetaMotor"
  HDL Subsystem/16(Iabc) -> Iabc/1  "Iabc"

== system m02_PMSM_HDL/FPGA Model/HDL Plant/Standard HDL Plant ==
  In1 : Inport
  Data Type Conversion : DataTypeConversion  SaturateOnIntegerOverflow=off  RndMeth=Floor
  Demux : Demux  Outputs=6
  HDL Subsystem : Subsystem
  thetaMotor : Outport
  omegaMotor : Outport  Port=2
  trqMotor : Outport  Port=3
  Iabc : Outport  Port=4
  wires:
  In1/1 -> Data Type Conversion/1
  HDL Subsystem/1(thetaMotor) -> thetaMotor/1  "thetaMotor"
  HDL Subsystem/2(omegaMotor) -> omegaMotor/1  "omegaMotor"
  HDL Subsystem/3(trqMotor) -> trqMotor/1  "trqMotor"
  HDL Subsystem/4(Iabc) -> Iabc/1  "Iabc"
  Demux/2 -> HDL Subsystem/2(GaL)
  Demux/3 -> HDL Subsystem/3(GbH)
  Demux/1 -> HDL Subsystem/1(GaH)
  Demux/4 -> HDL Subsystem/4(GbL)
  Demux/5 -> HDL Subsystem/5(GcH)
  Demux/6 -> HDL Subsystem/6(GcL)
  Data Type Conversion/1 -> Demux/1

== system m02_PMSM_HDL/FPGA Model/PWM Gate Signal Generator/HDL counter ==
  TgabcON : Inport
  TgabcOFF : Inport  Port=2
  Data Type Conversion : DataTypeConversion  SaturateOnIntegerOverflow=off  RndMeth=Floor
  Data Type Conversion1 : DataTypeConversion  SaturateOnIntegerOverflow=off  RndMeth=Floor
  Gain : Gain  Gain=Ts
  HDL Counter : hdlsllib/Sources/HDL Counter  CountType=Count limited  CountInit=0  CountStep=1  CountMax=floor(1/fsw/Ts-1)  CountFromType=Initial value  CountFrom=0  CountResetPort=off  CountLoadPort=off  CountEnbPort=off  CountDirPort=off  CountHitOutputPort=off  CountDataType=Unsigned  CountWordLen=16  CountFracLen=0  CountSampTime=Ts
  Logical Operator : Logic  Operator=XOR  AllPortsSameDT=off  OutDataTypeStr=boolean
  Logical Operator3 : Logic  Operator=NOT  AllPortsSameDT=off  OutDataTypeStr=boolean
  Mux : Mux  Inputs=2
  Relational Operator : RelationalOperator  OutDataTypeStr=boolean
  Relational Operator3 : RelationalOperator  OutDataTypeStr=boolean
  Selector : Selector  InputPortWidth=6  IndexOptions=Index vector (dialog)  Indices=[1 4 2 5 3 6]  OutputSizes=1
  g : Outport  VectorParamsAs1DForOutWhenUnconnected=off
  wires:
  Data Type Conversion/1 -> g/1
  Relational Operator/1 -> Logical Operator/1
  Logical Operator3/1 -> Mux/2
  Relational Operator3/1 -> Logical Operator/2
  TgabcOFF/1 -> Relational Operator3/2
  Logical Operator/1 -> Mux/1, Logical Operator3/1
  Selector/1 -> Data Type Conversion/1
  Gain/1 -> Relational Operator/1, Relational Operator3/1
  Mux/1 -> Selector/1
  TgabcON/1 -> Relational Operator/2
  HDL Counter/1 -> Data Type Conversion1/1
  Data Type Conversion1/1 -> Gain/1

== system m02_PMSM_HDL/PMSM controller/PMSM Field-Oriented Control/Inner loop control ==
  idq_ref : Inport
  wElectrical : Inport  Port=2
  iabc : Inport  Port=3
  theta : Inport  Port=4
  Vdc : Inport  Port=5
  Bias : Bias  Bias=theta_offset  SaturateOnIntegerOverflow=off
  Constant : Constant  Value=0  SampleTime=-1
  Gain : Gain  Gain=1/sqrt(3)
  PMSM Current Controller with Pre-Control : eePmsmCurrentController/PMSM Current Controller with Pre-Control  Kp_id=Kp_id  Ki_id=Ki_id  Kaw_id=Kaw_id  Kp_iq=Kp_iq  Ki_iq=Ki_iq  Kaw_iq=Kaw_iq  Ts=Tsc  Tsd=0.001  AxisPrio=Q-axis  ActZC=off  ActFF=on  idVect=idVect  iqVect=iqVect  LdMatrix=LdMatrix  LqMatrix=LqMatrix  psimMatrix=psimMatrix
  Park Transform : eeTransforms/Park Transform  AxisAlignment=Q-axis  PowerInvariant=off
  Selector : Selector  InputPortWidth=3  IndexOptions=Index vector (dialog)  Indices=[1 2]  OutputSizes=1
  vdqRef : Outport  VectorParamsAs1DForOutWhenUnconnected=off
  idq : Outport  Port=2  VectorParamsAs1DForOutWhenUnconnected=off
  wires:
  Bias/1 -> Park Transform/2
  PMSM Current Controller with Pre-Control/1 -> vdqRef/1
  Vdc/1 -> Gain/1
  wElectrical/1 -> PMSM Current Controller with Pre-Control/3
  theta/1 -> Bias/1
  iabc/1 -> Park Transform/1
  idq_ref/1 -> PMSM Current Controller with Pre-Control/1
  Park Transform/1 -> Selector/1
  Gain/1 -> PMSM Current Controller with Pre-Control/4
  Selector/1 -> idq/1, PMSM Current Controller with Pre-Control/2
  Constant/1 -> PMSM Current Controller with Pre-Control/5

== system m02_PMSM_HDL/PMSM controller/PMSM Field-Oriented Control/Input interface ==
  iabcSens : Inport
  wSens : Inport  Port=2
  thSens : Inport  Port=3
  VdcSens : Inport  Port=4
  2*pi : Constant  Value=2*pi  OutDataTypeStr=Inherit: Inherit via back propagation  SampleTime=Tsc
  Data Type Conversion Inherited : simulink/Signal Attributes/Data Type Conversion Inherited  ConvertRealWorld=Real World Value  DoSatur=off
  Math Function : Math  Operator=mod  SignedPower=on
  Relay : Relay  OnSwitchValue=Vdc_on  OffSwitchValue=0.5*Vdc_on
  pole pairs : Gain  Gain=p
  "pole pairs " : Gain  Gain=p
  wElectrical : Outport  VectorParamsAs1DForOutWhenUnconnected=off
  iabc : Outport  Port=2  VectorParamsAs1DForOutWhenUnconnected=off
  theta : Outport  Port=3  VectorParamsAs1DForOutWhenUnconnected=off
  Vdc : Outport  Port=4  VectorParamsAs1DForOutWhenUnconnected=off
  PwmEnable : Outport  Port=5  VectorParamsAs1DForOutWhenUnconnected=off
  wires:
  2*pi/1 -> Data Type Conversion Inherited/2
  Data Type Conversion Inherited/1 -> Math Function/2
  VdcSens/1 -> Vdc/1, Relay/1
  Relay/1 -> PwmEnable/1
  Math Function/1 -> theta/1
  "pole pairs "/1 -> Math Function/1, Data Type Conversion Inherited/1
  iabcSens/1 -> iabc/1
  wSens/1 -> pole pairs/1
  thSens/1 -> "pole pairs "/1
  pole pairs/1 -> wElectrical/1

== system m02_PMSM_HDL/PMSM controller/PMSM Field-Oriented Control/Outer loop control ==
  Reference : Inport
  wElectrical : Inport  Port=2
  Vdc : Inport  Port=3
  Constant : Constant  Value=0  OutDataTypeStr=Inherit: Inherit via back propagation  SampleTime=-1
  PMSM Current Reference Generator : eePmsmCurrentReferenceGen/PMSM Current Reference Generator  Vnom=Vnom  Pmax=Pmax  Tmax=Tmax  Ts=Tsc  RefType=Zero d-axis control  rpmVec=rpmVec  TqVec=TqVec  VdcVec=VdcVec  PWMMode=SPWM: sinusoidal PWM  ModFactor=ModFactor  idMatrix=idMatrix  iqMatrix=iqMatrix  p=p  psim=psim  Ld=Ld  Lq=Lq  Rs=Rs  RefExpEnable=0
  Tq Selector : Subsystem
  Velocity Controller : eeVelocityController/Velocity Controller  CtrlType=PI control  Kp_w=Kp_w  Ki_w=Ki_w  Kv_w=Kv_w  Kaw_w=Kaw_w  Ts=Tsc  Tsd=0.001  ActZC=off
  elec->mech : Gain  Gain=1/p
  idqRef : Outport  VectorParamsAs1DForOutWhenUnconnected=off
  TqRef : Outport  Port=2  VectorParamsAs1DForOutWhenUnconnected=off
  TqLim : Outport  Port=3  VectorParamsAs1DForOutWhenUnconnected=off
  wires:
  Velocity Controller/1 -> Tq Selector/2(TqRefUnsat)
  Tq Selector/1(TqRef) -> PMSM Current Reference Generator/1
  Constant/1 -> Velocity Controller/4
  elec->mech/1 -> Velocity Controller/2, PMSM Current Reference Generator/2
  PMSM Current Reference Generator/3 -> TqLim/1
  PMSM Current Reference Generator/2 -> TqRef/1, Velocity Controller/3
  PMSM Current Reference Generator/1 -> idqRef/1
  Vdc/1 -> PMSM Current Reference Generator/3
  wElectrical/1 -> elec->mech/1
  Reference/1 -> Tq Selector/1(Reference), Velocity Controller/1

== system m02_PMSM_HDL/PMSM controller/PMSM Field-Oriented Control/PWM ==
  vdqRef : Inport
  theta : Inport  Port=2
  Vdc : Inport  Port=3
  Constant : Constant  Value=0  SampleTime=Tsc
  Data Type Conversion Inherited : simulink/Signal Attributes/Data Type Conversion Inherited  ConvertRealWorld=Real World Value  DoSatur=off
  Inverse Park Transform : eeTransforms/Inverse Park Transform  AxisAlignment=Q-axis  PowerInvariant=off
  Mux : Mux  Inputs=2
  "PWM Generator (Three-phase, Two-level)" : Subsystem  AncestorBlock=|  LoadFcn=ee_sli_rtmsupport( 'loadfcn', gcbh );  mask(PWM Generator (three-phase, two-level)){PWMMode=Continuous PWM (CPWM), CPWMMode=SPWM: sinusoidal PWM, DPWMMode=60 DPWM: 60 degree discontinuous PWM, SamplingMode=Natural, fsw=fsw, Ts=Ts}
      | eePmsmFieldOrientedControl/PMSM Field-Oriented
      | Control/PWM/PWM Generator
      | (Three-phase, Two-level)
      mask prompts: PWMMode "physmod:ee:library:comments:control:eePwmGeneratorTwoLevel:PWMMode_MP"; CPWMMode "physmod:ee:library:comments:control:eePwmGeneratorTwoLevel:ContinuousPWM_MP"; DPWMMode "physmod:ee:library:comments:control:eePwmGeneratorTwoLevel:DiscontinuousPWM_MP"; SamplingMode "physmod:ee:library:comments:control:eePwmGeneratorTwoLevel:SamplingMode_MP"; fsw "physmod:ee:library:comments:control:eePwmGeneratorTwoLevel:SwitchingFrequencyHz_MP"; Ts "physmod:ee:library:comments:control:eePwmGeneratorTwoLevel:SampleTimes_MP"
      mask help: physmod:ee:library:comments:control:eePwmGeneratorTwoLevel:PWMGeneratorthreephaseTwolevel_MD
      mask init:
      | Tsw = 1/fsw;
      | 
      | if fsw <= 0
      |     error(message('physmod:simscape:compiler:patterns:checks:GreaterThanZero',getString(message('physmod:ee:library:comments:control:eePwmGeneratorTwoLevel:SwitchingFrequencyHz_MP'))));
      | end
      | 
      | if Ts <= 0
      |     error(message('physmod:simscape:compiler:patterns:checks:GreaterThanZero',getString(message('physmod:ee:library:comments:control:eePwmGeneratorTwoLevel:SampleTimes_MP'))));
      | end
      | 
      | if Ts > 1/(10*fsw)
      |     error(message('physmod:simscape:compiler:patterns:checks:LessThanOrEqual',getString(message('physmod:ee:library:comments:control:eePwmGeneratorTwoLevel:SampleTimes_MP')),getString(message('physmod:ee:library:comments:control:eePwmGeneratorTwoLevel:inverseOf10TimesSwitchingFrequency_MP'))));
      | end
      | 
      | switch SamplingMode
      |     case 'Natural'
      |         RateTransitionOnInput = -1;
      |         GateGeneratorX0 = 0;
      |     case 'Asymmetric'
      |         RateTransitionOnInput = 0.5*Tsw;
      |         GateGeneratorX0 = 0.5/fsw;
      |     case 'Symmetric'
      |         RateTransitionOnInput = Tsw;
      |         GateGeneratorX0 = 0;
      | end
      | 
      | 
      | switch PWMMode
      |     case 'Continuous PWM (CPWM)'
      |         switch CPWMMode
      |             case 'SPWM: sinusoidal PWM'
      |                 PWM = 1;
      |             case 'SVM: space vector modulation'
      |                 PWM = 2;
      |         end
      |     case 'Discontinuous PWM (DPWM)'
      |         switch DPWMMode
      |             case '60 DPWM: 60 degree discontinuous PWM'
      |                 PWM = 3;
      |             case '60 DPWM (+30 degree shift): +30 degree shift from 60 DPWM'
      |                 PWM = 4;
      |             case '60 DPWM (-30 degree shift): -30 degree shift from 60 DPWM'
      |                 PWM = 5;
      |             case '30 DPWM: 30 degree discontinuous PWM'
      |                 PWM = 6;
      |             case '120 DPWM: positive dc component'
      |                 PWM = 7;
      |             case '120 DPWM: negative dc component'
      |                 PWM = 8;
      |         end
      | end
      settings: CopyFcn=ee_sli_rtmsupport( 'copyfcn', gcbh );  DeleteFcn=ee_sli_rtmsupport( 'deletefcn', gcbh );  ModelCloseFcn=ee_sli_rtmsupport( 'modelclosefcn', gcbh );  PreSaveFcn=%pe_sli_rtmsupport( 'presavefcn', gcbh );  PostSaveFcn=ee_sli_rtmsupport( 'postsavefcn', gcbh );  PreCopyFcn=ee_sli_rtmsupport( 'precopyfcn', gcbh );  OpenFcn=ee_sli_rtmsupport( 'openfcn', gcbh );  CloseFcn=ee_sli_rtmsupport( 'closefcn', gcbh );  PreDeleteFcn=ee_sli_rtmsupport( 'predeletefcn', gcbh );
      mask Help: web(nesl_help(gcbh))
      mask TypeOptions PWMMode: physmod:ee:library:comments:control:eePwmGeneratorTwoLevel:ContinuousPWMCPWM_PV | physmod:ee:library:comments:control:eePwmGeneratorTwoLevel:DiscontinuousPWMDPWM_PV
      mask Callback PWMMode:
      | switch get_param(gcb,'PWMMode')
      |     case 'Continuous PWM (CPWM)'
      |         set_param(gcb,'MaskVisibilities',{'on';'on';'off';'on';'on';'on'})
      |     case 'Discontinuous PWM (DPWM)'
      |         set_param(gcb,'MaskVisibilities',{'on';'off';'on';'on';'on';'on'})
      | end
      mask TypeOptions CPWMMode: physmod:ee:library:comments:control:eePwmGeneratorTwoLevel:SPWMSinusoidalPWM_PV | physmod:ee:library:comments:control:eePwmGeneratorTwoLevel:SVMSpaceVectorModulation_PV
      mask TypeOptions DPWMMode: physmod:ee:library:comments:control:eePwmGeneratorTwoLevel:x60DPWM60DegreeDiscontinuousPWM_PV | physmod:ee:library:comments:control:eePwmGeneratorTwoLevel:x60DPWM30DegreeShift30DegreeShiftFrom60DPWM_PV | physmod:ee:library:comments:control:eePwmGeneratorTwoLevel:x60DPWM0x2D30DegreeShift0x2D30DegreeShiftFrom60DPWM_PV | physmod:ee:library:comments:control:eePwmGeneratorTwoLevel:x30DPWM30DegreeDiscontinuousPWM_PV | physmod:ee:library:comments:control:eePwmGeneratorTwoLevel:x120DPWMPositiveDcComponent_PV | physmod:ee:library:comments:control:eePwmGeneratorTwoLevel:x120DPWMNegativeDcComponent_PV
      mask TypeOptions SamplingMode: physmod:ee:library:comments:control:eePwmGeneratorTwoLevel:Natural_PV | physmod:ee:library:comments:control:eePwmGeneratorTwoLevel:Asymmetric_PV | physmod:ee:library:comments:control:eePwmGeneratorTwoLevel:Symmetric_PV
      mask DialogControl ParameterGroupVar Prompt: physmod:ee:library:comments:control:eePwmGeneratorTwoLevel:tab_Parameters
      mask DialogControl PWMMode Prompt: PWM mode
      mask DialogControl CPWMMode Prompt: Continuous PWM
      mask DialogControl DPWMMode Prompt: Discontinuous PWM
      mask DialogControl SamplingMode Prompt: Sampling mode
      mask DialogControl fsw Prompt: Switching frequency (Hz)
      mask DialogControl Ts Prompt: Sample time (s)
  TgabcON : Outport
  TgabcOFF : Outport  Port=2
  ModWave : Outport  Port=3  SampleTime=Tsc  VectorParamsAs1DForOutWhenUnconnected=off
  wires:
  Constant/1 -> Data Type Conversion Inherited/2
  Data Type Conversion Inherited/1 -> Mux/2
  Vdc/1 -> "PWM Generator (Three-phase, Two-level)"/2(vdc)
  Inverse Park Transform/1 -> "PWM Generator (Three-phase, Two-level)"/1(Vabc)
  "PWM Generator (Three-phase, Two-level)"/3(ModWave) -> ModWave/1
  Mux/1 -> Inverse Park Transform/1
  vdqRef/1 -> Mux/1, Data Type Conversion Inherited/1
  theta/1 -> Inverse Park Transform/2
  "PWM Generator (Three-phase, Two-level)"/1(TgabcON) -> TgabcON/1
  "PWM Generator (Three-phase, Two-level)"/2(TgabcOFF) -> TgabcOFF/1

== system m02_PMSM_HDL/FPGA Model/HDL Plant/Pejovic HDL Plant/HDL Subsystem ==
  ic_out2 : Inport
  ic_out4 : Inport  Port=2
  ic_out6 : Inport  Port=3
  ic_out1 : Inport  Port=4
  ic_out3 : Inport  Port=5
  ic_out5 : Inport  Port=6
  HDL Algorithm : Subsystem
  Input Concat : Concatenate  NumInputs=6
  Mux16 : Mux  Inputs=3
  Output Demux : Demux  Outputs=18
  thetaMotor : Outport
  omegaMotor : Outport  Port=2
  trqMotor : Outport  Port=3
  is_in1 : Outport  Port=4
  vs_in1 : Outport  Port=5
  is_in2 : Outport  Port=6
  vs_in2 : Outport  Port=7
  is_in3 : Outport  Port=8
  vs_in3 : Outport  Port=9
  is_in4 : Outport  Port=10
  vs_in4 : Outport  Port=11
  is_in5 : Outport  Port=12
  vs_in5 : Outport  Port=13
  is_in6 : Outport  Port=14
  vs_in6 : Outport  Port=15
  Iabc : Outport  Port=16
  wires:
  Output Demux/4 -> is_in1/1  "is_in1"
  HDL Algorithm/1(Out1) -> Output Demux/1
  Output Demux/18 -> Mux16/3
  Output Demux/11 -> vs_in4/1  "vs_in4"
  ic_out5/1 -> Input Concat/6
  ic_out3/1 -> Input Concat/5
  Output Demux/2 -> omegaMotor/1  "omegaMotor"
  Input Concat/1 -> HDL Algorithm/1(In1)
  Output Demux/17 -> Mux16/2
  Output Demux/15 -> vs_in6/1  "vs_in6"
  Output Demux/16 -> Mux16/1
  ic_out4/1 -> Input Concat/2
  ic_out6/1 -> Input Concat/3
  Output Demux/1 -> thetaMotor/1  "thetaMotor"
  ic_out1/1 -> Input Concat/4
  ic_out2/1 -> Input Concat/1
  Output Demux/7 -> vs_in2/1  "vs_in2"
  Output Demux/9 -> vs_in3/1  "vs_in3"
  Output Demux/3 -> trqMotor/1  "trqMotor"
  Output Demux/12 -> is_in5/1  "is_in5"
  Output Demux/6 -> is_in2/1  "is_in2"
  Output Demux/5 -> vs_in1/1  "vs_in1"
  Output Demux/10 -> is_in4/1  "is_in4"
  Output Demux/13 -> vs_in5/1  "vs_in5"
  Output Demux/8 -> is_in3/1  "is_in3"
  Output Demux/14 -> is_in6/1  "is_in6"
  Mux16/1 -> Iabc/1  "Iabc"

== system m02_PMSM_HDL/FPGA Model/HDL Plant/Standard HDL Plant/HDL Subsystem ==
  GaH : Inport
  GaL : Inport  Port=2
  GbH : Inport  Port=3
  GbL : Inport  Port=4
  GcH : Inport  Port=5
  GcL : Inport  Port=6
  HDL Algorithm : Subsystem
  Input Concat : Concatenate  NumInputs=6
  Mux4 : Mux  Inputs=3
  Output Demux : Demux  Outputs=6
  thetaMotor : Outport
  omegaMotor : Outport  Port=2
  trqMotor : Outport  Port=3
  Iabc : Outport  Port=4
  wires:
  HDL Algorithm/1(Out1) -> Output Demux/1
  Output Demux/4 -> Mux4/1
  Input Concat/1 -> HDL Algorithm/1(In1)
  GcH/1 -> Input Concat/5
  Output Demux/1 -> thetaMotor/1  "thetaMotor"
  Output Demux/6 -> Mux4/3
  Output Demux/5 -> Mux4/2
  GbL/1 -> Input Concat/4
  GcL/1 -> Input Concat/6
  GaH/1 -> Input Concat/1
  GbH/1 -> Input Concat/3
  GaL/1 -> Input Concat/2
  Output Demux/3 -> trqMotor/1  "trqMotor"
  Mux4/1 -> Iabc/1  "Iabc"
  Output Demux/2 -> omegaMotor/1  "omegaMotor"

== system m02_PMSM_HDL/PMSM controller/PMSM Field-Oriented Control/Outer loop control/Tq Selector ==
  Reference : Inport
  TqRefUnsat : Inport  Port=2
  Constant : Constant  Value=CtrlMode  SampleTime=Tsc
  Switch : Switch  Criteria=u2 > Threshold  Threshold=1.5  SaturateOnIntegerOverflow=off  InputSameDT=off
  TqRef : Outport  VectorParamsAs1DForOutWhenUnconnected=off
  wires:
  Switch/1 -> TqRef/1
  Constant/1 -> Switch/2
  TqRefUnsat/1 -> Switch/3
  Reference/1 -> Switch/1

== system m02_PMSM_HDL/PMSM controller/PMSM Field-Oriented Control/PWM/PWM Generator (Three-phase, Two-level) ==
  Vabc : Inport
  vdc : Inport  Port=2
  Data Type Conversion1 : DataTypeConversion  SaturateOnIntegerOverflow=off  RndMeth=Floor
  Data Type Conversion2 : DataTypeConversion  OutDataTypeStr=double  SaturateOnIntegerOverflow=off  RndMeth=Floor
  Data Type Conversion3 : DataTypeConversion  OutDataTypeStr=double  SaturateOnIntegerOverflow=off  RndMeth=Floor
  RTabc : RateTransition  OutPortSampleTime=RateTransitionOnInput
  RTdc : RateTransition  OutPortSampleTime=RateTransitionOnInput
  Switching Time Calculation : MATLAB Function  TreatAsAtomicUnit=on
  avoid division by 0 : Saturate  UpperLimit=inf  LowerLimit=eps
  TgabcON : Outport
  TgabcOFF : Outport  Port=2
  ModWave : Outport  Port=3  VectorParamsAs1DForOutWhenUnconnected=off
  wires:
  Data Type Conversion1/1 -> ModWave/1
  avoid division by 0/1 -> Switching Time Calculation/2(vdc)
  RTdc/1 -> avoid division by 0/1
  RTabc/1 -> Switching Time Calculation/1(Vabc)
  Switching Time Calculation/3(ModWave) -> Data Type Conversion1/1
  Switching Time Calculation/2(TgabcOFF) -> TgabcOFF/1
  Switching Time Calculation/1(TgabcON) -> TgabcON/1
  Vabc/1 -> Data Type Conversion2/1
  vdc/1 -> Data Type Conversion3/1
  Data Type Conversion2/1 -> RTabc/1
  Data Type Conversion3/1 -> RTdc/1

== system m02_PMSM_HDL/FPGA Model/HDL Plant/Pejovic HDL Plant/HDL Subsystem/HDL Algorithm ==
  In1 : Inport
  Clock : Subsystem
  Input Delay : Delay  DelayLength=1
  Output : Subsystem
  State Update : Subsystem
  t Delay : Delay  DelayLength=1
  Out1 : Outport  VectorParamsAs1DForOutWhenUnconnected=off
  wires:
  State Update/2(Mode) -> Output/4(Mode)
  Input Delay/1 -> Output/1(U)
  Clock/1(t) -> State Update/2(t), t Delay/1
  In1/1 -> State Update/1(U), Input Delay/1
  State Update/1(State) -> Output/2(State)
  t Delay/1 -> Output/3(t)
  Output/1(State Out) -> Out1/1

== system m02_PMSM_HDL/FPGA Model/HDL Plant/Standard HDL Plant/HDL Subsystem/HDL Algorithm ==
  In1 : Inport
  Clock : Subsystem
  Input Delay : Delay  DelayLength=1
  Output : Subsystem
  State Update : Subsystem
  t Delay : Delay  DelayLength=1
  Out1 : Outport  VectorParamsAs1DForOutWhenUnconnected=off
  wires:
  In1/1 -> State Update/1(U), Input Delay/1
  Output/1(State Out) -> Out1/1
  Input Delay/1 -> Output/1(U)
  Clock/1(t) -> State Update/2(t), t Delay/1
  State Update/2(Mode) -> Output/4(Mode)
  t Delay/1 -> Output/3(t)
  State Update/1(State) -> Output/2(State)

== system m02_PMSM_HDL/FPGA Model/HDL Plant/Pejovic HDL Plant/HDL Subsystem/HDL Algorithm/Clock ==
  Delay : Delay  DelayLength=1
  Sample Time : Constant  Value=single(2.5e-06)  OutDataTypeStr=single  SampleTime=2.5e-06
  Sum : Sum  OutDataTypeStr=single
  t : Outport  VectorParamsAs1DForOutWhenUnconnected=off
  wires:
  Sample Time/1 -> Sum/1
  Sum/1 -> Delay/1
  Delay/1 -> t/1, Sum/2
